simulink model "benchmark_model_2"  (R2021a)
settings: Solver=ode1  StartTime=0.0  StopTime=Tend  FixedStep=0.0001  MaxStep=0.1  MinStep=0.0001  AbsTol=0.01  EnableMultiTasking=on
values from neighbouring files (symbols this model uses):
  A1 = 0.00017774967488    [engine_data.mat]
  A2 = 740220.330082    [engine_data.mat]
  AL = [6 6.5 7 7.5 8 8.5 9 9.5 10 10.5 11 11.5 ... (33 elements, 33x1)]    [engine_data.mat]
  AM0 = 0.02884    [engine_data.mat]
  AREA = 0.00580880481649    [engine_data.mat]
  BORE = 0.086    [engine_data.mat]
  C_EGR = 1.5    [engine_data.mat]
  c_f = 800000    [engine_data.mat]
  c_T = 1    [engine_data.mat]
  CAIR = [0 0 0 0.21 0 0 0.79]    [engine_data.mat]
  cCO = 0    [engine_data.mat]
  cCO2 = 0    [engine_data.mat]
  cH2 = 0    [engine_data.mat]
  cH2O = 0    [engine_data.mat]
  cHC = 0    [engine_data.mat]
  cN2 = 0.79    [engine_data.mat]
  CO = [22.3416398376 20.8398063107 19.3759939408 17.9445472871 16.538827802 15.1528221174 13.7819470707 12.4234138404 11.076283262 9.74128071245 8.42044156849 7.11667724438 ... (33 elements, 33x1)]    [engine_data.mat]
  CO2 = [1.08016197936 1.63070203699 2.20578946805 2.80905596198 3.44329822989 4.11013545224 4.80975559522 5.54078746844 6.30033629562 7.08419123341 7.88717005398 8.70352822078 ... (33 elements, 33x1)]    [engine_data.mat]
  cO2 = 0.21    [engine_data.mat]
  DEN0 = 1.17881164668    [engine_data.mat]
  EGR_dia = 0.02    [engine_data.mat]
  EGR_sk = 0.125663706144    [engine_data.mat]
  EX_AREA = 0.00137444678595    [engine_data.mat]
  EX_M_AR = 0.0258532162804    [engine_data.mat]
  EXO = 40    [engine_data.mat]
  FD0 = 5    [engine_data.mat]
  FOM = [12 11.348 6.233 5 5.449 8.523 5]    [engine_data.mat]
  FR0 = 0    [engine_data.mat]
  FR_C1 = 305.731    [engine_data.mat]
  FR_C2 = 1.70183    [engine_data.mat]
  FR_C3 = 3188.7424    [engine_data.mat]
  FR_C4 = 0.000296028194151    [engine_data.mat]
  FR_C5 = 1.03    [engine_data.mat]
  H2 = [17.3855302766 15.0102176452 12.8820660449 10.9850020715 9.30240027035 7.81790027685 6.51548255669 5.37933989743 4.39378660966 3.5433012035 2.8127075229 2.1874445405 ... (33 elements, 33x1)]    [engine_data.mat]
  H2O = [3.81120036781 5.32559240945 6.64944794012 7.79700886885 8.78142378855 9.61507632366 10.310008356 10.8782622871 11.3320540899 11.6837509075 11.9456809954 12.1298414055 ... (33 elements, 33x1)]    [engine_data.mat]
  HC = [5481.3024964 4476.06435729 3754.34247414 3215.30411383 2799.83726136 2471.30975971 2205.97110777 1987.83348465 1805.78690133 1651.89669698 1520.35918152 1406.8402103 ... (33 elements, 33x1)]    [engine_data.mat]
  INC = 0    [engine_data.mat]
  INO = -40    [engine_data.mat]
  KET = 0.001    [engine_data.mat]
  Kex = 1.28224854645    [engine_data.mat]
  Kh = 0.00462    [engine_data.mat]
  MAS0 = 0.00471524658673    [engine_data.mat]
  MCh = 0.000588883862304    [engine_data.mat]
  MHC = 0.01383448    [engine_data.mat]
  MN2 = 0.028    [engine_data.mat]
  MO2 = 0.032    [engine_data.mat]
  MOLcylT = 0.00157069204711    [engine_data.mat]
  N2 = [54.5020363032 56.4529864816 58.2465252261 59.8999246568 61.4284172656 62.8453054261 64.1621746691 65.3891205654 66.5349581592 67.6074047194 68.6132342687 69.5584035698 ... (33 elements, 33x1)]    [engine_data.mat]
  O2 = [0.331300985803 0.293088680307 0.264743132617 0.242930742419 0.225648917415 0.211629427842 0.200034641439 0.190292592782 0.182002893523 0.174881554044 0.168729672297 0.163420998081 ... (33 elements, 33x1)]    [engine_data.mat]
  PR0 = 101324.72    [engine_data.mat]
  R150 = 157.079632679    [engine_data.mat]
  Rabs = 8.31441    [engine_data.mat]
  SPEC = [4 0.086 0.086 0.043 0.14665 14 1 0.1 0 0.5 0.005 0 ... (19 elements, 19x1)]    [engine_data.mat]
  TBORE = 0.055    [engine_data.mat]
  Tend = 120    [engine_data.mat]
  Th_HC = 0.1    [engine_data.mat]
  Th_knock = 0.401961937891    [engine_data.mat]
  THEX = [0 1 2 3 4 5 6 7 8 9 10 11 ... (721 elements, 1x721)]    [engine_data.mat]
  THIN = [0 1 2 3 4 5 6 7 8 9 10 11 ... (721 elements, 1x721)]    [engine_data.mat]
  TM0 = 298.15    [engine_data.mat]
  Tstart = 5    [engine_data.mat]
  TW0 = 353.15    [engine_data.mat]
  V_EX = 0.0001    [engine_data.mat]
  VAREX = [0 0 0 0 0 0 0 0 0 0 0 0 ... (721 elements, 1x721)]    [engine_data.mat]
  VARIN = [0 0 0 0 0 0 0 0 0 0 0 0 ... (721 elements, 1x721)]    [engine_data.mat]
  VH = 0.000499557214218    [engine_data.mat]
  VT = 3.84274780168e-05    [engine_data.mat]
  WOM = [0.01383448 0.04401 0.02801 0.032 0.002016 0.018016 0.028]    [engine_data.mat]
  y = 1.81    [engine_data.mat]
undefined symbols (not defined in the file or in its folder): DiscIntNeverNeededParam
libraries: pid_lib x3
(part 2 of 7)

== system benchmark_model_2/ENGINE/engine_s/cylinders/cyl3 ==
  In_state : Inport
  In_c : Inport  Port=2
  ex_state : Inport  Port=3
  ex_c : Inport  Port=4
  ECU_sa : Inport  Port=5
  ECU_fi : Inport  Port=6
  rps : Inport  Port=7
  st : Inport  Port=8
  EGR : Inport  Port=9
  in_vt : Inport  Port=10
  cyl : Subsystem
  ex_valve : Subsystem
  in_valve : Subsystem
  selectors : Subsystem
  af : Outport
  ex_fen : Outport  Port=2
  ex_fml : Outport  Port=3
  in_fen : Outport  Port=4
  in_fml : Outport  Port=5
  pc : Outport  Port=6
  QA : Outport  Port=7
  QR : Outport  Port=8
  KI : Outport  Port=9
  Knock : Outport  Port=10
  RHC : Outport  Port=11
  TR : Outport  Port=12
  sum_fc : Outport  Port=13
  fc : Outport  Port=14
  wires:
  rps/1 -> cyl/7(rps), selectors/7(rps)
  ECU_fi/1 -> selectors/6(ECU_fi)
  ECU_sa/1 -> selectors/5(ECU_sa)
  st/1 -> selectors/4(st)
  In_state/1 -> in_valve/5(u_st)
  ex_state/1 -> ex_valve/1(d_st)
  cyl/1(cyl_state) -> in_valve/2(d_st), ex_valve/4(u_st)
  cyl/2(cyl_c) -> ex_valve/5(u_c), in_valve/1(d_c)
  In_c/1 -> in_valve/6(u_c)
  selectors/1(ecu) -> ex_valve/3(ecu), in_valve/3(ecu), cyl/5(ecu)
  cyl/3(pc) -> pc/1
  ex_c/1 -> ex_valve/2(d_c)
  ex_valve/1(fen) -> cyl/1(ex_fen), ex_fen/1
  ex_valve/2(fml) -> cyl/2(ex_fml), ex_fml/1
  in_valve/1(fen) -> cyl/3(in_fen), in_fen/1
  in_valve/2(fml) -> cyl/4(in_fml), selectors/1(fml), in_fml/1
  cyl/4(af) -> af/1
  selectors/2(KL) -> cyl/6(KL)
  cyl/5(QA) -> QA/1
  cyl/6(QR) -> QR/1
  cyl/7(KI) -> KI/1
  in_valve/3(fms) -> selectors/2(fms)
  EGR/1 -> cyl/8(EGR)
  cyl/8(Knock) -> Knock/1
  cyl/9(R_HC) -> RHC/1
  in_vt/1 -> selectors/3(ECU_vt), in_valve/4(in_vt)
  cyl/10(TR) -> TR/1
  selectors/3(sum_fc) -> sum_fc/1
  selectors/4(fc) -> fc/1

== system benchmark_model_2/ENGINE/engine_s/cylinders/cyl4 ==
  In_state : Inport
  In_c : Inport  Port=2
  ex_state : Inport  Port=3
  ex_c : Inport  Port=4
  ECU_sa : Inport  Port=5
  ECU_fi : Inport  Port=6
  rps : Inport  Port=7
  st : Inport  Port=8
  EGR : Inport  Port=9
  in_vt : Inport  Port=10
  cyl : Subsystem
  ex_valve : Subsystem
  in_valve : Subsystem
  selectors : Subsystem
  af : Outport
  ex_fen : Outport  Port=2
  ex_fml : Outport  Port=3
  in_fen : Outport  Port=4
  in_fml : Outport  Port=5
  pc : Outport  Port=6
  QA : Outport  Port=7
  QR : Outport  Port=8
  KI : Outport  Port=9
  Knock : Outport  Port=10
  RHC : Outport  Port=11
  TR : Outport  Port=12
  sum_fc : Outport  Port=13
  fc : Outport  Port=14
  wires:
  selectors/3(sum_fc) -> sum_fc/1
  cyl/10(TR) -> TR/1
  in_vt/1 -> in_valve/4(in_vt), selectors/3(ECU_vt)
  cyl/9(R_HC) -> RHC/1
  cyl/8(Knock) -> Knock/1
  EGR/1 -> cyl/8(EGR)
  in_valve/3(fms) -> selectors/2(fms)
  cyl/7(KI) -> KI/1
  cyl/6(QR) -> QR/1
  cyl/5(QA) -> QA/1
  selectors/2(KL) -> cyl/6(KL)
  cyl/4(af) -> af/1
  in_valve/2(fml) -> in_fml/1, selectors/1(fml), cyl/4(in_fml)
  in_valve/1(fen) -> in_fen/1, cyl/3(in_fen)
  ex_valve/2(fml) -> ex_fml/1, cyl/2(ex_fml)
  ex_valve/1(fen) -> ex_fen/1, cyl/1(ex_fen)
  ex_c/1 -> ex_valve/2(d_c)
  cyl/3(pc) -> pc/1
  selectors/1(ecu) -> cyl/5(ecu), in_valve/3(ecu), ex_valve/3(ecu)
  In_c/1 -> in_valve/6(u_c)
  cyl/2(cyl_c) -> in_valve/1(d_c), ex_valve/5(u_c)
  cyl/1(cyl_state) -> ex_valve/4(u_st), in_valve/2(d_st)
  ex_state/1 -> ex_valve/1(d_st)
  In_state/1 -> in_valve/5(u_st)
  st/1 -> selectors/4(st)
  ECU_sa/1 -> selectors/5(ECU_sa)
  ECU_fi/1 -> selectors/6(ECU_fi)
  rps/1 -> selectors/7(rps), cyl/7(rps)
  selectors/4(fc) -> fc/1

== system benchmark_model_2/ENGINE/engine_s/ex_chamber/In_vol ==
  EGR_fen : Inport
  EGR_fml : Inport  Port=2
  out_fen : Inport  Port=3
  out_fml : Inport  Port=4
  in_fen : Inport  Port=5
  in_fml : Inport  Port=6
  Enrgy_Int : Subsystem
  Mol_Int : Subsystem
  cal_cyl_state : Subsystem
  V_temp : Outport  InitialOutput=0
  V_state : Outport  Port=2  InitialOutput=0
  V_c : Outport  Port=3  InitialOutput=0
  wires:
  cal_cyl_state/1(V_temp) -> Enrgy_Int/1(temp), V_temp/1
  out_fen/1 -> Enrgy_Int/3(Enrgy_out)
  in_fen/1 -> Enrgy_Int/2(Enrgy_In)
  out_fml/1 -> Mol_Int/2(nml_out)
  in_fml/1 -> Mol_Int/1(nml_In)
  Enrgy_Int/1(E) -> cal_cyl_state/1(E)
  Mol_Int/1(Nmol) -> cal_cyl_state/2(Nml)
  cal_cyl_state/2(V_st) -> V_state/1
  cal_cyl_state/3(V_c) -> V_c/1
  EGR_fen/1 -> Enrgy_Int/4(Enrgy_EGR)
  EGR_fml/1 -> Mol_Int/3(nml_EGR)

== system benchmark_model_2/ENGINE/engine_s/in_chamber/In_vol ==
  EGR_fen : Inport
  EGR_fml : Inport  Port=2
  out_fen : Inport  Port=3
  out_fml : Inport  Port=4
  in_fen : Inport  Port=5
  in_fml : Inport  Port=6
  Enrgy_Int : Subsystem
  Mol_Int : Subsystem
  cal_cyl_state : Subsystem
  C_signed_C : Outport  InitialOutput=0
  V_state : Outport  Port=2  InitialOutput=0
  V_c : Outport  Port=3  InitialOutput=0
  C_C : Outport  Port=4  InitialOutput=0
  wires:
  cal_cyl_state/2(V_c) -> V_c/1
  cal_cyl_state/1(V_st) -> V_state/1
  Mol_Int/1(Nmol) -> cal_cyl_state/2(Nml)
  Enrgy_Int/1(X_dens) -> cal_cyl_state/1(E)
  in_fml/1 -> Mol_Int/1(nml_In)
  out_fml/1 -> Mol_Int/2(nml_out)
  in_fen/1 -> Enrgy_Int/1(Enrgy_In)
  out_fen/1 -> Enrgy_Int/2(Enrgy_out)
  EGR_fen/1 -> Enrgy_Int/3(Enrgy_EGR)
  EGR_fml/1 -> Mol_Int/3(nml_EGR)
  Mol_Int/2(C_signed_C) -> C_signed_C/1
  Mol_Int/3(C_C) -> C_C/1

== system benchmark_model_2/ENGINE/engine_s/rpm_dynamics1/stroke ==
  CA : Inport
  Constant : Constant  Value=pi
  Mux : Mux
  Sum : Sum  Inputs=+-|  InputSameDT=on  SaturateOnIntegerOverflow=on  OutDataTypeStr=Inherit: Same as first input
  Sum1 : Sum  Inputs=+-|  InputSameDT=on  SaturateOnIntegerOverflow=on  OutDataTypeStr=Inherit: Same as first input
  Sum2 : Sum  Inputs=+-|  InputSameDT=on  SaturateOnIntegerOverflow=on  OutDataTypeStr=Inherit: Same as first input
  mod720(u,4*pi) : Subsystem
  mod720(u,4*pi)1 : Subsystem
  mod720(u,4*pi)2 : Subsystem
  mod720(u,4*pi)3 : Subsystem
  st(1-4) : Outport
  wires:
  CA/1 -> mod720(u,4*pi)/1(u), Sum/1
  mod720(u,4*pi)/1(y) -> Mux/1
  Mux/1 -> st(1-4)/1
  Sum2/1 -> mod720(u,4*pi)3/1(u)
  Constant/1 -> Sum1/2, Sum/2, Sum2/2
  Sum1/1 -> mod720(u,4*pi)2/1(u), Sum2/1
  Sum/1 -> mod720(u,4*pi)1/1(u), Sum1/1
  mod720(u,4*pi)1/1(y) -> Mux/3
  mod720(u,4*pi)2/1(y) -> Mux/4
  mod720(u,4*pi)3/1(y) -> Mux/2

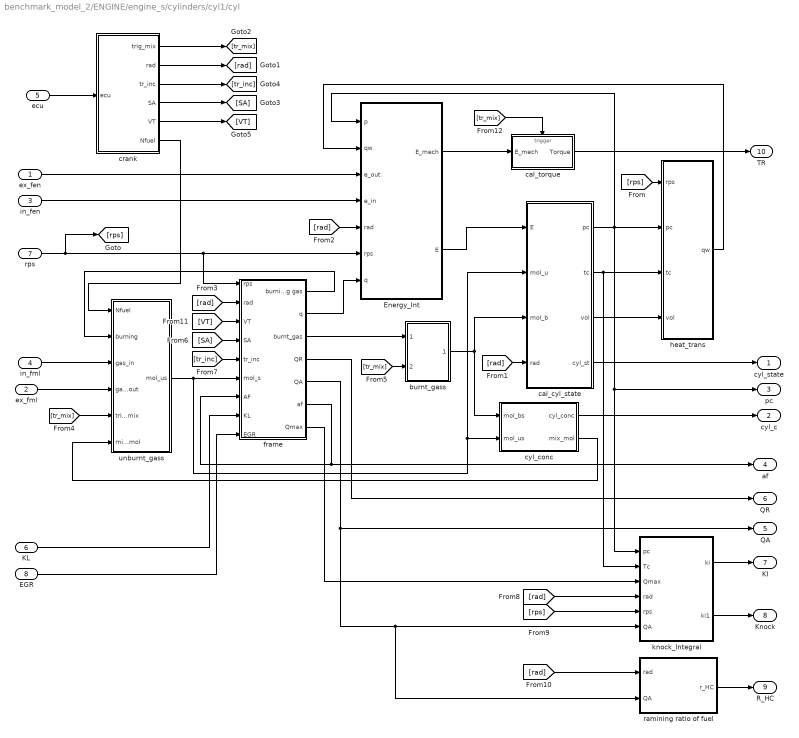
== system benchmark_model_2/ENGINE/engine_s/cylinders/cyl1/cyl ==
  ex_fen : Inport
  ex_fml : Inport  Port=2
  in_fen : Inport  Port=3
  in_fml : Inport  Port=4
  ecu : Inport  Port=5
  KL : Inport  Port=6
  rps : Inport  Port=7
  EGR : Inport  Port=8
  Energy_Int : Subsystem
  burnt_gass : Subsystem
  cal_cyl_state : Subsystem
  cal_torque : Subsystem
  crank : Subsystem
  cyl_conc : Subsystem
  frame : Subsystem
  heat_trans : Subsystem
  knock_Integral : Subsystem
  ramining ratio of fuel : Subsystem
  unburnt_gass : Subsystem
  cyl_state : Outport  InitialOutput=0
  cyl_c : Outport  Port=2  InitialOutput=0
  pc : Outport  Port=3  InitialOutput=0
  af : Outport  Port=4  InitialOutput=0
  QA : Outport  Port=5  InitialOutput=0
  QR : Outport  Port=6  InitialOutput=0
  KI : Outport  Port=7  InitialOutput=0
  Knock : Outport  Port=8  InitialOutput=0
  R_HC : Outport  Port=9  InitialOutput=0
  TR : Outport  Port=10  InitialOutput=0
  wires:
  heat_trans/1(qw) -> Energy_Int/2(qw)
  frame/2(q) -> Energy_Int/7(q)
  frame/3(burnt_gas) -> burnt_gass/1(gas_in)
  unburnt_gass/1(mol_us) -> cyl_conc/2(mol_us), cal_cyl_state/2(mol_u), frame/6(mol_s)
  rps/1 -> [rps], frame/1(rps), Energy_Int/6(rps)
  in_fml/1 -> unburnt_gass/3(gas_in)
  burnt_gass/1(mol_bs) -> cal_cyl_state/3(mol_b), cyl_conc/1(mol_bs)
  cyl_conc/1(cyl_conc) -> cyl_c/1
  [rps] -> heat_trans/1(rps)
  ecu/1 -> crank/1(ecu)
  [rad] -> Energy_Int/5(rad)
  [rad] -> frame/2(rad)
  ex_fen/1 -> Energy_Int/3(e_out)
  in_fen/1 -> Energy_Int/4(e_in)
  ex_fml/1 -> unburnt_gass/4(gas_out)
  frame/1(burning gas) -> unburnt_gass/2(burning)
  crank/1(trig_mix) -> [tr_mix]
  [tr_mix] -> unburnt_gass/5(trig_mix)
  [tr_mix] -> burnt_gass/2(tr_mix)
  crank/2(rad) -> [rad]
  frame/6(af) -> af/1, frame/7(AF)
  crank/6(Nfuel) -> unburnt_gass/1(Nfuel)
  [tr_inc] -> frame/5(tr_inc)
  cyl_conc/2(mix_mol) -> unburnt_gass/6(mix_mol)
  crank/3(tr_inc) -> [tr_inc]
  cal_cyl_state/1(pc) -> heat_trans/2(pc), Energy_Int/1(p), pc/1, knock_Integral/1(pc)
  [rad] -> cal_cyl_state/4(rad)
  cal_cyl_state/4(cyl_st) -> cyl_state/1
  cal_cyl_state/3(vol) -> heat_trans/4(vol)
  cal_cyl_state/2(tc) -> knock_Integral/2(Tc), heat_trans/3(tc)
  Energy_Int/2(E) -> cal_cyl_state/1(E)
  crank/4(SA) -> [SA]
  [SA] -> frame/4(SA)
  KL/1 -> frame/8(KL)
  frame/4(QR) -> QR/1
  knock_Integral/1(ki) -> KI/1
  EGR/1 -> frame/9(EGR)
  [rad] -> knock_Integral/4(rad)
  frame/5(QA) -> QA/1, ramining ratio of fuel/2(QA), knock_Integral/6(QA)
  [rps] -> knock_Integral/5(rps)
  knock_Integral/2(ki1) -> Knock/1
  [rad] -> ramining ratio of fuel/1(rad)
  ramining ratio of fuel/1(r_HC) -> R_HC/1
  frame/7(Qmax) -> knock_Integral/3(Qmax)
  [VT] -> frame/3(VT)
  crank/5(VT) -> [VT]
  Energy_Int/1(E_mech) -> cal_torque/1(E_mech)
  cal_torque/1(Torque) -> TR/1
  [tr_mix] -> cal_torque/Trigger

== system benchmark_model_2/ENGINE/engine_s/cylinders/cyl1/ex_valve ==
  d_st : Inport
  d_c : Inport  Port=2
  ecu : Inport  Port=3
  u_st : Inport  Port=4  PortDimensions=4
  u_c : Inport  Port=5
  Constant : Constant  Value=WOM
  Constant1 : Constant  Value=4*pi
  Gain : Gain  Gain=180/pi
  Lookup Table1 : Lookup  InputValues=THEX  Table=VAREX
  Math Function : Math  Operator=mod  SignedPower=on  SaturateOnIntegerOverflow=on
  Selector : Selector  InputPortWidth=6  IndexOptions=Index vector (dialog)  Indices=1  OutputSizes=[(-2)]
  cal_flow : MATLAB Function  TreatAsAtomicUnit=on
  fen : Outport  PortDimensions=1
  fml : Outport  Port=2  PortDimensions=7
  wires:
  ecu/1 -> Selector/1
  cal_flow/1(fen) -> fen/1
  Lookup Table1/1 -> cal_flow/1(area)
  u_st/1 -> cal_flow/2(inlet)
  u_c/1 -> cal_flow/3(c_in)
  d_st/1 -> cal_flow/4(outlet)
  d_c/1 -> cal_flow/5(c_out)
  cal_flow/2(fml) -> fml/1
  Constant/1 -> cal_flow/6(WOM)
  Gain/1 -> Lookup Table1/1
  Math Function/1 -> Gain/1
  Selector/1 -> Math Function/1
  Constant1/1 -> Math Function/2

== system benchmark_model_2/ENGINE/engine_s/cylinders/cyl1/in_valve ==
  d_c : Inport
  d_st : Inport  Port=2
  ecu : Inport  Port=3
  in_vt : Inport  Port=4
  u_st : Inport  Port=5
  u_c : Inport  Port=6
  Add : Sum  Inputs=-+
  Constant : Constant  Value=WOM
  Gain : Gain  Gain=180/pi
  Lookup Table : Lookup  InputValues=THIN  Table=VARIN
  Selector1 : Selector  InputPortWidth=6  IndexOptions=Index vector (dialog)  Indices=1  OutputSizes=[(-2)]
  cal_flow : MATLAB Function  TreatAsAtomicUnit=on
  fen : Outport  PortDimensions=1
  fml : Outport  Port=2  PortDimensions=7
  fms : Outport  Port=3  PortDimensions=1
  wires:
  Gain/1 -> Lookup Table/1
  ecu/1 -> Selector1/1
  u_st/1 -> cal_flow/2(inlet)
  Lookup Table/1 -> cal_flow/1(area)
  d_st/1 -> cal_flow/4(outlet)
  cal_flow/1(fen) -> fen/1
  u_c/1 -> cal_flow/3(c_in)
  d_c/1 -> cal_flow/5(c_out)
  cal_flow/2(fml) -> fml/1
  cal_flow/3(fms) -> fms/1
  Constant/1 -> cal_flow/6(WOM)
  in_vt/1 -> Add/1
  Selector1/1 -> Add/2
  Add/1 -> Gain/1

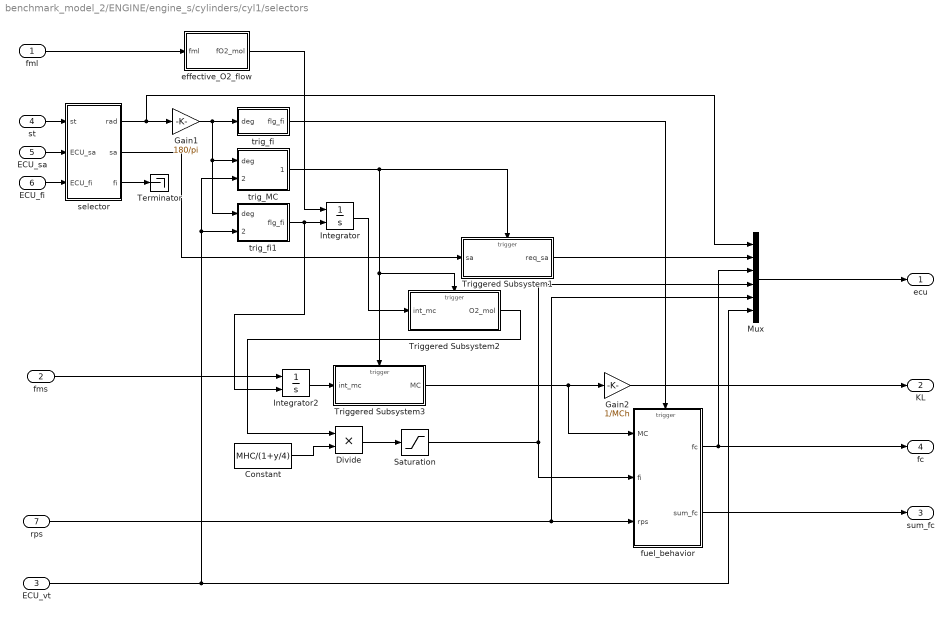
== system benchmark_model_2/ENGINE/engine_s/cylinders/cyl1/selectors ==
  fml : Inport
  fms : Inport  Port=2
  ECU_vt : Inport  Port=3
  st : Inport  Port=4
  ECU_sa : Inport  Port=5
  ECU_fi : Inport  Port=6
  rps : Inport  Port=7
  Constant : Constant  Value=MHC/(1+y/4)
  Divide : Product
  Gain1 : Gain  Gain=180/pi
  Gain2 : Gain  Gain=1/MCh
  Integrator : Integrator  ExternalReset=rising
  Integrator2 : Integrator  ExternalReset=rising
  Mux : Mux  Inputs=6
  Saturation : Saturate  UpperLimit=inf  LowerLimit=0
  Terminator : Terminator
  Triggered Subsystem1 : Subsystem  TreatAsAtomicUnit=on
  Triggered Subsystem2 : Subsystem  TreatAsAtomicUnit=on
  Triggered Subsystem3 : Subsystem  TreatAsAtomicUnit=on
  effective_O2_flow : Subsystem
  fuel_behavior : Subsystem  TreatAsAtomicUnit=on
  selector : Subsystem
  trig_MC : Subsystem
  trig_fi : Subsystem
  trig_fi1 : Subsystem
  ecu : Outport
  KL : Outport  Port=2
  sum_fc : Outport  Port=3
  fc : Outport  Port=4
  wires:
  Triggered Subsystem2/1(O2_mol) -> Divide/1
  Gain1/1 -> trig_fi/1(deg), trig_fi1/1(deg), trig_MC/1(deg)
  ECU_fi/1 -> selector/3(ECU_fi)
  ECU_sa/1 -> selector/2(ECU_sa)
  st/1 -> selector/1(st)
  trig_MC/1(flg_inc) -> Triggered Subsystem3/Trigger, Triggered Subsystem2/Trigger, Triggered Subsystem1/Trigger
  rps/1 -> Mux/5, fuel_behavior/3(rps)
  selector/1(rad) -> Gain1/1, Mux/1
  Mux/1 -> ecu/1
  trig_fi/1(flg_fi) -> fuel_behavior/Trigger
  selector/2(sa) -> Triggered Subsystem1/1(sa)
  Triggered Subsystem1/1(req_sa) -> Mux/2
  trig_fi1/1(flg_fi) -> Integrator/2, Integrator2/2
  Integrator/1 -> Triggered Subsystem2/1(int_mc)
  fuel_behavior/1(fc) -> fc/1, Mux/3
  selector/3(fi) -> Terminator/1
  Gain2/1 -> KL/1
  Divide/1 -> Saturation/1
  fml/1 -> effective_O2_flow/1(fml)
  effective_O2_flow/1(fO2_mol) -> Integrator/1
  Constant/1 -> Divide/2
  Saturation/1 -> fuel_behavior/2(fi), Mux/4
  Integrator2/1 -> Triggered Subsystem3/1(int_mc)
  Triggered Subsystem3/1(MC) -> Gain2/1, fuel_behavior/1(MC)
  fms/1 -> Integrator2/1
  ECU_vt/1 -> trig_MC/2(ECU_vvt), trig_fi1/2(ECU_vvt), Mux/6
  fuel_behavior/2(sum_fc) -> sum_fc/1

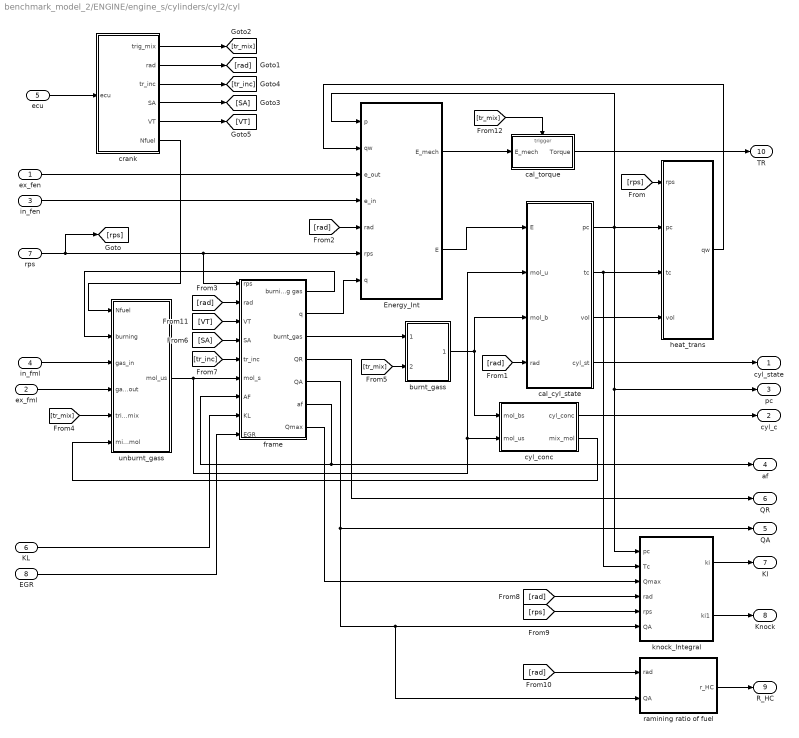
== system benchmark_model_2/ENGINE/engine_s/cylinders/cyl2/cyl ==
  ex_fen : Inport
  ex_fml : Inport  Port=2
  in_fen : Inport  Port=3
  in_fml : Inport  Port=4
  ecu : Inport  Port=5
  KL : Inport  Port=6
  rps : Inport  Port=7
  EGR : Inport  Port=8
  Energy_Int : Subsystem
  burnt_gass : Subsystem
  cal_cyl_state : Subsystem
  cal_torque : Subsystem
  crank : Subsystem
  cyl_conc : Subsystem
  frame : Subsystem
  heat_trans : Subsystem
  knock_Integral : Subsystem
  ramining ratio of fuel : Subsystem
  unburnt_gass : Subsystem
  cyl_state : Outport  InitialOutput=0
  cyl_c : Outport  Port=2  InitialOutput=0
  pc : Outport  Port=3  InitialOutput=0
  af : Outport  Port=4  InitialOutput=0
  QA : Outport  Port=5  InitialOutput=0
  QR : Outport  Port=6  InitialOutput=0
  KI : Outport  Port=7  InitialOutput=0
  Knock : Outport  Port=8  InitialOutput=0
  R_HC : Outport  Port=9  InitialOutput=0
  TR : Outport  Port=10  InitialOutput=0
  wires:
  [tr_mix] -> cal_torque/Trigger
  cal_torque/1(Torque) -> TR/1
  Energy_Int/1(E_mech) -> cal_torque/1(E_mech)
  crank/5(VT) -> [VT]
  [VT] -> frame/3(VT)
  frame/7(Qmax) -> knock_Integral/3(Qmax)
  ramining ratio of fuel/1(r_HC) -> R_HC/1
  [rad] -> ramining ratio of fuel/1(rad)
  knock_Integral/2(ki1) -> Knock/1
  [rps] -> knock_Integral/5(rps)
  frame/5(QA) -> knock_Integral/6(QA), ramining ratio of fuel/2(QA), QA/1
  [rad] -> knock_Integral/4(rad)
  EGR/1 -> frame/9(EGR)
  knock_Integral/1(ki) -> KI/1
  frame/4(QR) -> QR/1
  KL/1 -> frame/8(KL)
  [SA] -> frame/4(SA)
  crank/4(SA) -> [SA]
  Energy_Int/2(E) -> cal_cyl_state/1(E)
  cal_cyl_state/2(tc) -> heat_trans/3(tc), knock_Integral/2(Tc)
  cal_cyl_state/3(vol) -> heat_trans/4(vol)
  cal_cyl_state/4(cyl_st) -> cyl_state/1
  [rad] -> cal_cyl_state/4(rad)
  cal_cyl_state/1(pc) -> knock_Integral/1(pc), pc/1, Energy_Int/1(p), heat_trans/2(pc)
  crank/3(tr_inc) -> [tr_inc]
  cyl_conc/2(mix_mol) -> unburnt_gass/6(mix_mol)
  [tr_inc] -> frame/5(tr_inc)
  crank/6(Nfuel) -> unburnt_gass/1(Nfuel)
  frame/6(af) -> frame/7(AF), af/1
  crank/2(rad) -> [rad]
  [tr_mix] -> burnt_gass/2(tr_mix)
  [tr_mix] -> unburnt_gass/5(trig_mix)
  crank/1(trig_mix) -> [tr_mix]
  frame/1(burning gas) -> unburnt_gass/2(burning)
  ex_fml/1 -> unburnt_gass/4(gas_out)
  in_fen/1 -> Energy_Int/4(e_in)
  ex_fen/1 -> Energy_Int/3(e_out)
  [rad] -> frame/2(rad)
  [rad] -> Energy_Int/5(rad)
  ecu/1 -> crank/1(ecu)
  [rps] -> heat_trans/1(rps)
  cyl_conc/1(cyl_conc) -> cyl_c/1
  burnt_gass/1(mol_bs) -> cyl_conc/1(mol_bs), cal_cyl_state/3(mol_b)
  in_fml/1 -> unburnt_gass/3(gas_in)
  rps/1 -> Energy_Int/6(rps), frame/1(rps), [rps]
  unburnt_gass/1(mol_us) -> frame/6(mol_s), cal_cyl_state/2(mol_u), cyl_conc/2(mol_us)
  frame/3(burnt_gas) -> burnt_gass/1(gas_in)
  frame/2(q) -> Energy_Int/7(q)
  heat_trans/1(qw) -> Energy_Int/2(qw)

== system benchmark_model_2/ENGINE/engine_s/cylinders/cyl2/ex_valve ==
  d_st : Inport
  d_c : Inport  Port=2
  ecu : Inport  Port=3
  u_st : Inport  Port=4  PortDimensions=4
  u_c : Inport  Port=5
  Constant : Constant  Value=WOM
  Constant1 : Constant  Value=4*pi
  Gain : Gain  Gain=180/pi
  Lookup Table1 : Lookup  InputValues=THEX  Table=VAREX
  Math Function : Math  Operator=mod  SignedPower=on  SaturateOnIntegerOverflow=on
  Selector : Selector  InputPortWidth=6  IndexOptions=Index vector (dialog)  Indices=1  OutputSizes=[(-2)]
  cal_flow : MATLAB Function  TreatAsAtomicUnit=on
  fen : Outport  PortDimensions=1
  fml : Outport  Port=2  PortDimensions=7
  wires:
  Constant1/1 -> Math Function/2
  Selector/1 -> Math Function/1
  Math Function/1 -> Gain/1
  Gain/1 -> Lookup Table1/1
  Constant/1 -> cal_flow/6(WOM)
  cal_flow/2(fml) -> fml/1
  d_c/1 -> cal_flow/5(c_out)
  d_st/1 -> cal_flow/4(outlet)
  u_c/1 -> cal_flow/3(c_in)
  u_st/1 -> cal_flow/2(inlet)
  Lookup Table1/1 -> cal_flow/1(area)
  cal_flow/1(fen) -> fen/1
  ecu/1 -> Selector/1

== system benchmark_model_2/ENGINE/engine_s/cylinders/cyl2/in_valve ==
  d_c : Inport
  d_st : Inport  Port=2
  ecu : Inport  Port=3
  in_vt : Inport  Port=4
  u_st : Inport  Port=5
  u_c : Inport  Port=6
  Add : Sum  Inputs=-+
  Constant : Constant  Value=WOM
  Gain : Gain  Gain=180/pi
  Lookup Table : Lookup  InputValues=THIN  Table=VARIN
  Selector1 : Selector  InputPortWidth=6  IndexOptions=Index vector (dialog)  Indices=1  OutputSizes=[(-2)]
  cal_flow : MATLAB Function  TreatAsAtomicUnit=on
  fen : Outport  PortDimensions=1
  fml : Outport  Port=2  PortDimensions=7
  fms : Outport  Port=3  PortDimensions=1
  wires:
  Add/1 -> Gain/1
  Selector1/1 -> Add/2
  in_vt/1 -> Add/1
  Constant/1 -> cal_flow/6(WOM)
  cal_flow/3(fms) -> fms/1
  cal_flow/2(fml) -> fml/1
  d_c/1 -> cal_flow/5(c_out)
  u_c/1 -> cal_flow/3(c_in)
  cal_flow/1(fen) -> fen/1
  d_st/1 -> cal_flow/4(outlet)
  Lookup Table/1 -> cal_flow/1(area)
  u_st/1 -> cal_flow/2(inlet)
  ecu/1 -> Selector1/1
  Gain/1 -> Lookup Table/1

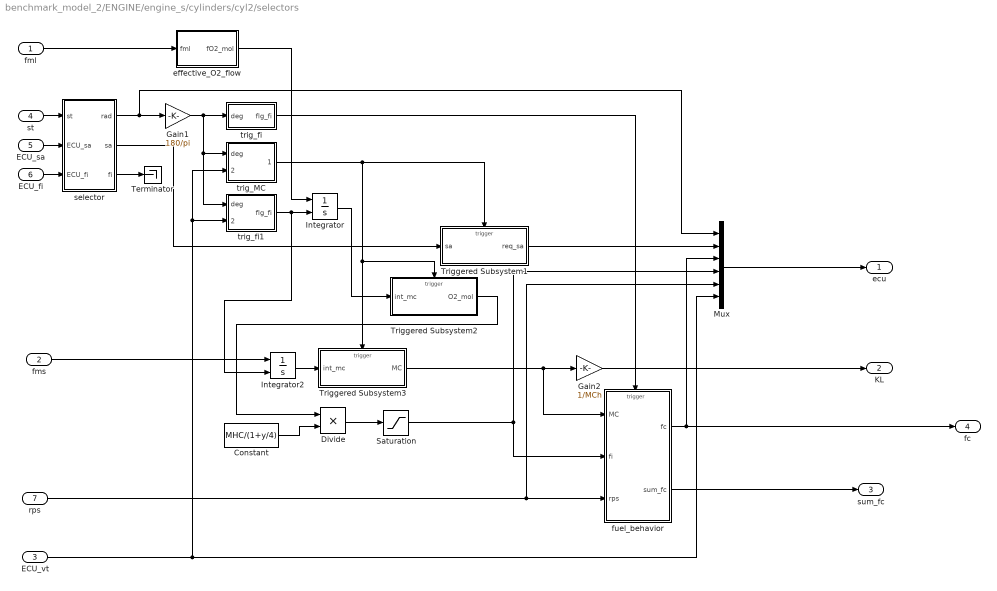
== system benchmark_model_2/ENGINE/engine_s/cylinders/cyl2/selectors ==
  fml : Inport
  fms : Inport  Port=2
  ECU_vt : Inport  Port=3
  st : Inport  Port=4
  ECU_sa : Inport  Port=5
  ECU_fi : Inport  Port=6
  rps : Inport  Port=7
  Constant : Constant  Value=MHC/(1+y/4)
  Divide : Product
  Gain1 : Gain  Gain=180/pi
  Gain2 : Gain  Gain=1/MCh
  Integrator : Integrator  ExternalReset=rising
  Integrator2 : Integrator  ExternalReset=rising
  Mux : Mux  Inputs=6
  Saturation : Saturate  UpperLimit=inf  LowerLimit=0
  Terminator : Terminator
  Triggered Subsystem1 : Subsystem  TreatAsAtomicUnit=on
  Triggered Subsystem2 : Subsystem  TreatAsAtomicUnit=on
  Triggered Subsystem3 : Subsystem  TreatAsAtomicUnit=on
  effective_O2_flow : Subsystem
  fuel_behavior : Subsystem  TreatAsAtomicUnit=on
  selector : Subsystem
  trig_MC : Subsystem
  trig_fi : Subsystem
  trig_fi1 : Subsystem
  ecu : Outport
  KL : Outport  Port=2
  sum_fc : Outport  Port=3
  fc : Outport  Port=4
  wires:
  fuel_behavior/2(sum_fc) -> sum_fc/1
  ECU_vt/1 -> Mux/6, trig_fi1/2(ECU_vvt), trig_MC/2(ECU_vvt)
  fms/1 -> Integrator2/1
  Triggered Subsystem3/1(MC) -> fuel_behavior/1(MC), Gain2/1
  Integrator2/1 -> Triggered Subsystem3/1(int_mc)
  Saturation/1 -> Mux/4, fuel_behavior/2(fi)
  Constant/1 -> Divide/2
  effective_O2_flow/1(fO2_mol) -> Integrator/1
  fml/1 -> effective_O2_flow/1(fml)
  Divide/1 -> Saturation/1
  Gain2/1 -> KL/1
  selector/3(fi) -> Terminator/1
  Integrator/1 -> Triggered Subsystem2/1(int_mc)
  trig_fi1/1(flg_fi) -> Integrator2/2, Integrator/2
  Triggered Subsystem1/1(req_sa) -> Mux/2
  selector/2(sa) -> Triggered Subsystem1/1(sa)
  trig_fi/1(flg_fi) -> fuel_behavior/Trigger
  Mux/1 -> ecu/1
  selector/1(rad) -> Mux/1, Gain1/1
  rps/1 -> fuel_behavior/3(rps), Mux/5
  trig_MC/1(flg_inc) -> Triggered Subsystem1/Trigger, Triggered Subsystem2/Trigger, Triggered Subsystem3/Trigger
  st/1 -> selector/1(st)
  ECU_sa/1 -> selector/2(ECU_sa)
  ECU_fi/1 -> selector/3(ECU_fi)
  Gain1/1 -> trig_MC/1(deg), trig_fi1/1(deg), trig_fi/1(deg)
  Triggered Subsystem2/1(O2_mol) -> Divide/1
  fuel_behavior/1(fc) -> fc/1, Mux/3

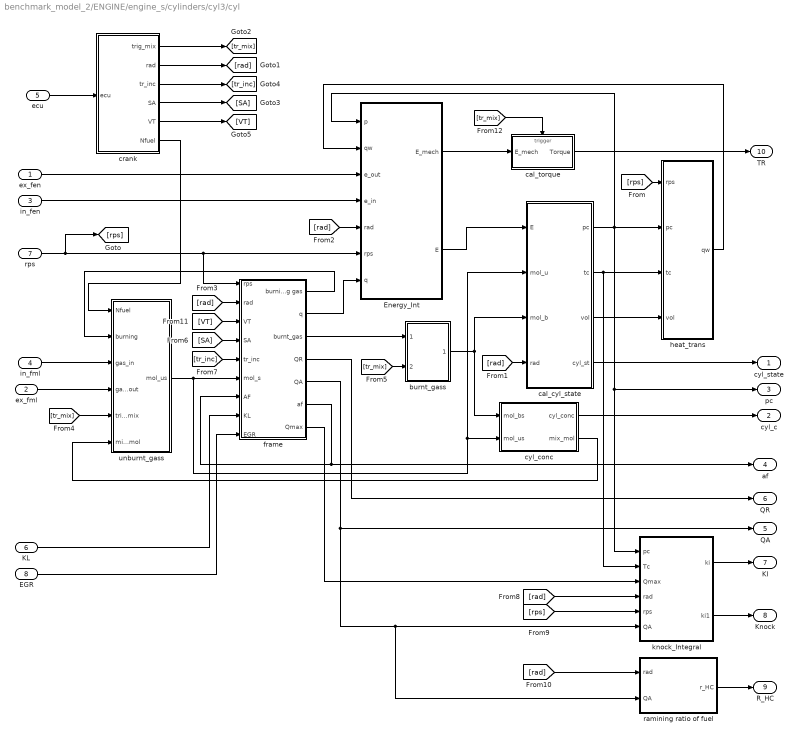
== system benchmark_model_2/ENGINE/engine_s/cylinders/cyl3/cyl ==
  ex_fen : Inport
  ex_fml : Inport  Port=2
  in_fen : Inport  Port=3
  in_fml : Inport  Port=4
  ecu : Inport  Port=5
  KL : Inport  Port=6
  rps : Inport  Port=7
  EGR : Inport  Port=8
  Energy_Int : Subsystem
  burnt_gass : Subsystem
  cal_cyl_state : Subsystem
  cal_torque : Subsystem
  crank : Subsystem
  cyl_conc : Subsystem
  frame : Subsystem
  heat_trans : Subsystem
  knock_Integral : Subsystem
  ramining ratio of fuel : Subsystem
  unburnt_gass : Subsystem
  cyl_state : Outport  InitialOutput=0
  cyl_c : Outport  Port=2  InitialOutput=0
  pc : Outport  Port=3  InitialOutput=0
  af : Outport  Port=4  InitialOutput=0
  QA : Outport  Port=5  InitialOutput=0
  QR : Outport  Port=6  InitialOutput=0
  KI : Outport  Port=7  InitialOutput=0
  Knock : Outport  Port=8  InitialOutput=0
  R_HC : Outport  Port=9  InitialOutput=0
  TR : Outport  Port=10  InitialOutput=0
  wires:
  heat_trans/1(qw) -> Energy_Int/2(qw)
  frame/2(q) -> Energy_Int/7(q)
  frame/3(burnt_gas) -> burnt_gass/1(gas_in)
  unburnt_gass/1(mol_us) -> cyl_conc/2(mol_us), cal_cyl_state/2(mol_u), frame/6(mol_s)
  rps/1 -> [rps], frame/1(rps), Energy_Int/6(rps)
  in_fml/1 -> unburnt_gass/3(gas_in)
  burnt_gass/1(mol_bs) -> cal_cyl_state/3(mol_b), cyl_conc/1(mol_bs)
  cyl_conc/1(cyl_conc) -> cyl_c/1
  [rps] -> heat_trans/1(rps)
  ecu/1 -> crank/1(ecu)
  [rad] -> Energy_Int/5(rad)
  [rad] -> frame/2(rad)
  ex_fen/1 -> Energy_Int/3(e_out)
  in_fen/1 -> Energy_Int/4(e_in)
  ex_fml/1 -> unburnt_gass/4(gas_out)
  frame/1(burning gas) -> unburnt_gass/2(burning)
  crank/1(trig_mix) -> [tr_mix]
  [tr_mix] -> unburnt_gass/5(trig_mix)
  [tr_mix] -> burnt_gass/2(tr_mix)
  crank/2(rad) -> [rad]
  frame/6(af) -> af/1, frame/7(AF)
  crank/6(Nfuel) -> unburnt_gass/1(Nfuel)
  [tr_inc] -> frame/5(tr_inc)
  cyl_conc/2(mix_mol) -> unburnt_gass/6(mix_mol)
  crank/3(tr_inc) -> [tr_inc]
  cal_cyl_state/1(pc) -> heat_trans/2(pc), Energy_Int/1(p), pc/1, knock_Integral/1(pc)
  [rad] -> cal_cyl_state/4(rad)
  cal_cyl_state/4(cyl_st) -> cyl_state/1
  cal_cyl_state/3(vol) -> heat_trans/4(vol)
  cal_cyl_state/2(tc) -> knock_Integral/2(Tc), heat_trans/3(tc)
  Energy_Int/2(E) -> cal_cyl_state/1(E)
  crank/4(SA) -> [SA]
  [SA] -> frame/4(SA)
  KL/1 -> frame/8(KL)
  frame/4(QR) -> QR/1
  knock_Integral/1(ki) -> KI/1
  EGR/1 -> frame/9(EGR)
  [rad] -> knock_Integral/4(rad)
  frame/5(QA) -> QA/1, ramining ratio of fuel/2(QA), knock_Integral/6(QA)
  [rps] -> knock_Integral/5(rps)
  knock_Integral/2(ki1) -> Knock/1
  [rad] -> ramining ratio of fuel/1(rad)
  ramining ratio of fuel/1(r_HC) -> R_HC/1
  frame/7(Qmax) -> knock_Integral/3(Qmax)
  [VT] -> frame/3(VT)
  crank/5(VT) -> [VT]
  Energy_Int/1(E_mech) -> cal_torque/1(E_mech)
  cal_torque/1(Torque) -> TR/1
  [tr_mix] -> cal_torque/Trigger

== system benchmark_model_2/ENGINE/engine_s/cylinders/cyl3/ex_valve ==
  d_st : Inport
  d_c : Inport  Port=2
  ecu : Inport  Port=3
  u_st : Inport  Port=4  PortDimensions=4
  u_c : Inport  Port=5
  Constant : Constant  Value=WOM
  Constant1 : Constant  Value=4*pi
  Gain : Gain  Gain=180/pi
  Lookup Table1 : Lookup  InputValues=THEX  Table=VAREX
  Math Function : Math  Operator=mod  SignedPower=on  SaturateOnIntegerOverflow=on
  Selector : Selector  InputPortWidth=6  IndexOptions=Index vector (dialog)  Indices=1  OutputSizes=[(-2)]
  cal_flow : MATLAB Function  TreatAsAtomicUnit=on
  fen : Outport  PortDimensions=1
  fml : Outport  Port=2  PortDimensions=7
  wires:
  ecu/1 -> Selector/1
  cal_flow/1(fen) -> fen/1
  Lookup Table1/1 -> cal_flow/1(area)
  u_st/1 -> cal_flow/2(inlet)
  u_c/1 -> cal_flow/3(c_in)
  d_st/1 -> cal_flow/4(outlet)
  d_c/1 -> cal_flow/5(c_out)
  cal_flow/2(fml) -> fml/1
  Constant/1 -> cal_flow/6(WOM)
  Gain/1 -> Lookup Table1/1
  Math Function/1 -> Gain/1
  Selector/1 -> Math Function/1
  Constant1/1 -> Math Function/2

== system benchmark_model_2/ENGINE/engine_s/cylinders/cyl3/in_valve ==
  d_c : Inport
  d_st : Inport  Port=2
  ecu : Inport  Port=3
  in_vt : Inport  Port=4
  u_st : Inport  Port=5
  u_c : Inport  Port=6
  Add : Sum  Inputs=-+
  Constant : Constant  Value=WOM
  Gain : Gain  Gain=180/pi
  Lookup Table : Lookup  InputValues=THIN  Table=VARIN
  Selector1 : Selector  InputPortWidth=6  IndexOptions=Index vector (dialog)  Indices=1  OutputSizes=[(-2)]
  cal_flow : MATLAB Function  TreatAsAtomicUnit=on
  fen : Outport  PortDimensions=1
  fml : Outport  Port=2  PortDimensions=7
  fms : Outport  Port=3  PortDimensions=1
  wires:
  Gain/1 -> Lookup Table/1
  ecu/1 -> Selector1/1
  u_st/1 -> cal_flow/2(inlet)
  Lookup Table/1 -> cal_flow/1(area)
  d_st/1 -> cal_flow/4(outlet)
  cal_flow/1(fen) -> fen/1
  u_c/1 -> cal_flow/3(c_in)
  d_c/1 -> cal_flow/5(c_out)
  cal_flow/2(fml) -> fml/1
  cal_flow/3(fms) -> fms/1
  Constant/1 -> cal_flow/6(WOM)
  in_vt/1 -> Add/1
  Selector1/1 -> Add/2
  Add/1 -> Gain/1

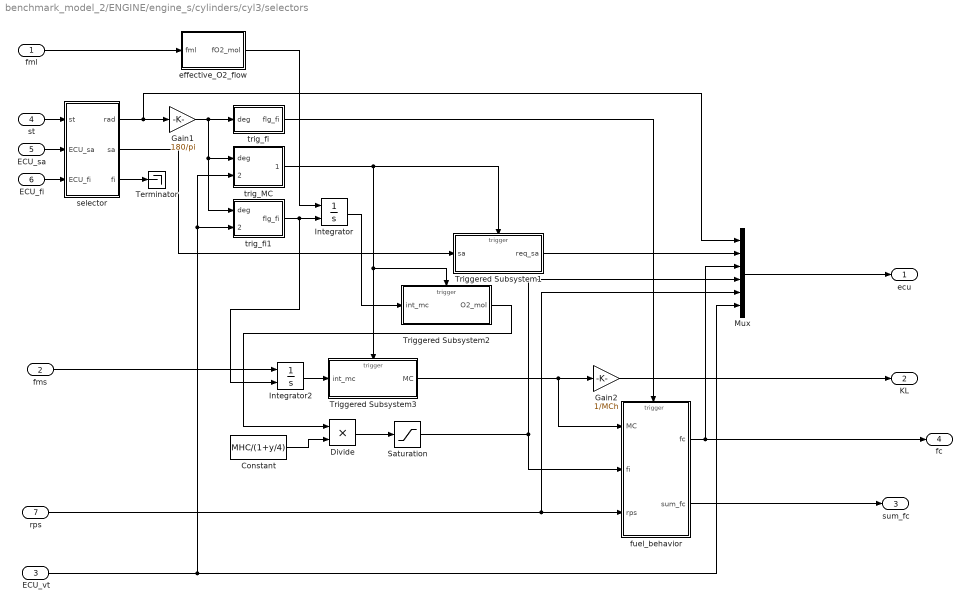
== system benchmark_model_2/ENGINE/engine_s/cylinders/cyl3/selectors ==
  fml : Inport
  fms : Inport  Port=2
  ECU_vt : Inport  Port=3
  st : Inport  Port=4
  ECU_sa : Inport  Port=5
  ECU_fi : Inport  Port=6
  rps : Inport  Port=7
  Constant : Constant  Value=MHC/(1+y/4)
  Divide : Product
  Gain1 : Gain  Gain=180/pi
  Gain2 : Gain  Gain=1/MCh
  Integrator : Integrator  ExternalReset=rising
  Integrator2 : Integrator  ExternalReset=rising
  Mux : Mux  Inputs=6
  Saturation : Saturate  UpperLimit=inf  LowerLimit=0
  Terminator : Terminator
  Triggered Subsystem1 : Subsystem  TreatAsAtomicUnit=on
  Triggered Subsystem2 : Subsystem  TreatAsAtomicUnit=on
  Triggered Subsystem3 : Subsystem  TreatAsAtomicUnit=on
  effective_O2_flow : Subsystem
  fuel_behavior : Subsystem  TreatAsAtomicUnit=on
  selector : Subsystem
  trig_MC : Subsystem
  trig_fi : Subsystem
  trig_fi1 : Subsystem
  ecu : Outport
  KL : Outport  Port=2
  sum_fc : Outport  Port=3
  fc : Outport  Port=4
  wires:
  Triggered Subsystem2/1(O2_mol) -> Divide/1
  Gain1/1 -> trig_fi/1(deg), trig_fi1/1(deg), trig_MC/1(deg)
  ECU_fi/1 -> selector/3(ECU_fi)
  ECU_sa/1 -> selector/2(ECU_sa)
  st/1 -> selector/1(st)
  trig_MC/1(flg_inc) -> Triggered Subsystem3/Trigger, Triggered Subsystem2/Trigger, Triggered Subsystem1/Trigger
  rps/1 -> Mux/5, fuel_behavior/3(rps)
  selector/1(rad) -> Gain1/1, Mux/1
  Mux/1 -> ecu/1
  trig_fi/1(flg_fi) -> fuel_behavior/Trigger
  selector/2(sa) -> Triggered Subsystem1/1(sa)
  Triggered Subsystem1/1(req_sa) -> Mux/2
  trig_fi1/1(flg_fi) -> Integrator/2, Integrator2/2
  Integrator/1 -> Triggered Subsystem2/1(int_mc)
  selector/3(fi) -> Terminator/1
  Gain2/1 -> KL/1
  Divide/1 -> Saturation/1
  fml/1 -> effective_O2_flow/1(fml)
  effective_O2_flow/1(fO2_mol) -> Integrator/1
  Constant/1 -> Divide/2
  Saturation/1 -> fuel_behavior/2(fi), Mux/4
  Integrator2/1 -> Triggered Subsystem3/1(int_mc)
  Triggered Subsystem3/1(MC) -> Gain2/1, fuel_behavior/1(MC)
  fms/1 -> Integrator2/1
  ECU_vt/1 -> trig_MC/2(ECU_vvt), trig_fi1/2(ECU_vvt), Mux/6
  fuel_behavior/2(sum_fc) -> sum_fc/1
  fuel_behavior/1(fc) -> fc/1, Mux/3

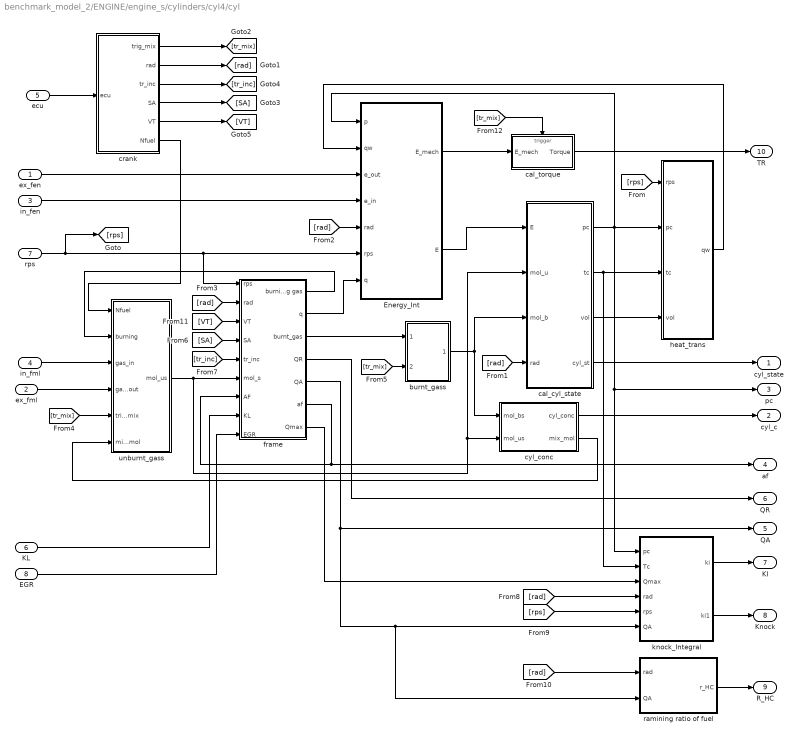
== system benchmark_model_2/ENGINE/engine_s/cylinders/cyl4/cyl ==
  ex_fen : Inport
  ex_fml : Inport  Port=2
  in_fen : Inport  Port=3
  in_fml : Inport  Port=4
  ecu : Inport  Port=5
  KL : Inport  Port=6
  rps : Inport  Port=7
  EGR : Inport  Port=8
  Energy_Int : Subsystem
  burnt_gass : Subsystem
  cal_cyl_state : Subsystem
  cal_torque : Subsystem
  crank : Subsystem
  cyl_conc : Subsystem
  frame : Subsystem
  heat_trans : Subsystem
  knock_Integral : Subsystem
  ramining ratio of fuel : Subsystem
  unburnt_gass : Subsystem
  cyl_state : Outport  InitialOutput=0
  cyl_c : Outport  Port=2  InitialOutput=0
  pc : Outport  Port=3  InitialOutput=0
  af : Outport  Port=4  InitialOutput=0
  QA : Outport  Port=5  InitialOutput=0
  QR : Outport  Port=6  InitialOutput=0
  KI : Outport  Port=7  InitialOutput=0
  Knock : Outport  Port=8  InitialOutput=0
  R_HC : Outport  Port=9  InitialOutput=0
  TR : Outport  Port=10  InitialOutput=0
  wires:
  [tr_mix] -> cal_torque/Trigger
  cal_torque/1(Torque) -> TR/1
  Energy_Int/1(E_mech) -> cal_torque/1(E_mech)
  crank/5(VT) -> [VT]
  [VT] -> frame/3(VT)
  frame/7(Qmax) -> knock_Integral/3(Qmax)
  ramining ratio of fuel/1(r_HC) -> R_HC/1
  [rad] -> ramining ratio of fuel/1(rad)
  knock_Integral/2(ki1) -> Knock/1
  [rps] -> knock_Integral/5(rps)
  frame/5(QA) -> knock_Integral/6(QA), ramining ratio of fuel/2(QA), QA/1
  [rad] -> knock_Integral/4(rad)
  EGR/1 -> frame/9(EGR)
  knock_Integral/1(ki) -> KI/1
  frame/4(QR) -> QR/1
  KL/1 -> frame/8(KL)
  [SA] -> frame/4(SA)
  crank/4(SA) -> [SA]
  Energy_Int/2(E) -> cal_cyl_state/1(E)
  cal_cyl_state/2(tc) -> heat_trans/3(tc), knock_Integral/2(Tc)
  cal_cyl_state/3(vol) -> heat_trans/4(vol)
  cal_cyl_state/4(cyl_st) -> cyl_state/1
  [rad] -> cal_cyl_state/4(rad)
  cal_cyl_state/1(pc) -> knock_Integral/1(pc), pc/1, Energy_Int/1(p), heat_trans/2(pc)
  crank/3(tr_inc) -> [tr_inc]
  cyl_conc/2(mix_mol) -> unburnt_gass/6(mix_mol)
  [tr_inc] -> frame/5(tr_inc)
  crank/6(Nfuel) -> unburnt_gass/1(Nfuel)
  frame/6(af) -> frame/7(AF), af/1
  crank/2(rad) -> [rad]
  [tr_mix] -> burnt_gass/2(tr_mix)
  [tr_mix] -> unburnt_gass/5(trig_mix)
  crank/1(trig_mix) -> [tr_mix]
  frame/1(burning gas) -> unburnt_gass/2(burning)
  ex_fml/1 -> unburnt_gass/4(gas_out)
  in_fen/1 -> Energy_Int/4(e_in)
  ex_fen/1 -> Energy_Int/3(e_out)
  [rad] -> frame/2(rad)
  [rad] -> Energy_Int/5(rad)
  ecu/1 -> crank/1(ecu)
  [rps] -> heat_trans/1(rps)
  cyl_conc/1(cyl_conc) -> cyl_c/1
  burnt_gass/1(mol_bs) -> cyl_conc/1(mol_bs), cal_cyl_state/3(mol_b)
  in_fml/1 -> unburnt_gass/3(gas_in)
  rps/1 -> Energy_Int/6(rps), frame/1(rps), [rps]
  unburnt_gass/1(mol_us) -> frame/6(mol_s), cal_cyl_state/2(mol_u), cyl_conc/2(mol_us)
  frame/3(burnt_gas) -> burnt_gass/1(gas_in)
  frame/2(q) -> Energy_Int/7(q)
  heat_trans/1(qw) -> Energy_Int/2(qw)

== system benchmark_model_2/ENGINE/engine_s/cylinders/cyl4/ex_valve ==
  d_st : Inport
  d_c : Inport  Port=2
  ecu : Inport  Port=3
  u_st : Inport  Port=4  PortDimensions=4
  u_c : Inport  Port=5
  Constant : Constant  Value=WOM
  Constant1 : Constant  Value=4*pi
  Gain : Gain  Gain=180/pi
  Lookup Table1 : Lookup  InputValues=THEX  Table=VAREX
  Math Function : Math  Operator=mod  SignedPower=on  SaturateOnIntegerOverflow=on
  Selector : Selector  InputPortWidth=6  IndexOptions=Index vector (dialog)  Indices=1  OutputSizes=[(-2)]
  cal_flow : MATLAB Function  TreatAsAtomicUnit=on
  fen : Outport  PortDimensions=1
  fml : Outport  Port=2  PortDimensions=7
  wires:
  Constant1/1 -> Math Function/2
  Selector/1 -> Math Function/1
  Math Function/1 -> Gain/1
  Gain/1 -> Lookup Table1/1
  Constant/1 -> cal_flow/6(WOM)
  cal_flow/2(fml) -> fml/1
  d_c/1 -> cal_flow/5(c_out)
  d_st/1 -> cal_flow/4(outlet)
  u_c/1 -> cal_flow/3(c_in)
  u_st/1 -> cal_flow/2(inlet)
  Lookup Table1/1 -> cal_flow/1(area)
  cal_flow/1(fen) -> fen/1
  ecu/1 -> Selector/1

== system benchmark_model_2/ENGINE/engine_s/cylinders/cyl4/in_valve ==
  d_c : Inport
  d_st : Inport  Port=2
  ecu : Inport  Port=3
  in_vt : Inport  Port=4
  u_st : Inport  Port=5
  u_c : Inport  Port=6
  Add : Sum  Inputs=-+
  Constant : Constant  Value=WOM
  Gain : Gain  Gain=180/pi
  Lookup Table : Lookup  InputValues=THIN  Table=VARIN
  Selector1 : Selector  InputPortWidth=6  IndexOptions=Index vector (dialog)  Indices=1  OutputSizes=[(-2)]
  cal_flow : MATLAB Function  TreatAsAtomicUnit=on
  fen : Outport  PortDimensions=1
  fml : Outport  Port=2  PortDimensions=7
  fms : Outport  Port=3  PortDimensions=1
  wires:
  Add/1 -> Gain/1
  Selector1/1 -> Add/2
  in_vt/1 -> Add/1
  Constant/1 -> cal_flow/6(WOM)
  cal_flow/3(fms) -> fms/1
  cal_flow/2(fml) -> fml/1
  d_c/1 -> cal_flow/5(c_out)
  u_c/1 -> cal_flow/3(c_in)
  cal_flow/1(fen) -> fen/1
  d_st/1 -> cal_flow/4(outlet)
  Lookup Table/1 -> cal_flow/1(area)
  u_st/1 -> cal_flow/2(inlet)
  ecu/1 -> Selector1/1
  Gain/1 -> Lookup Table/1

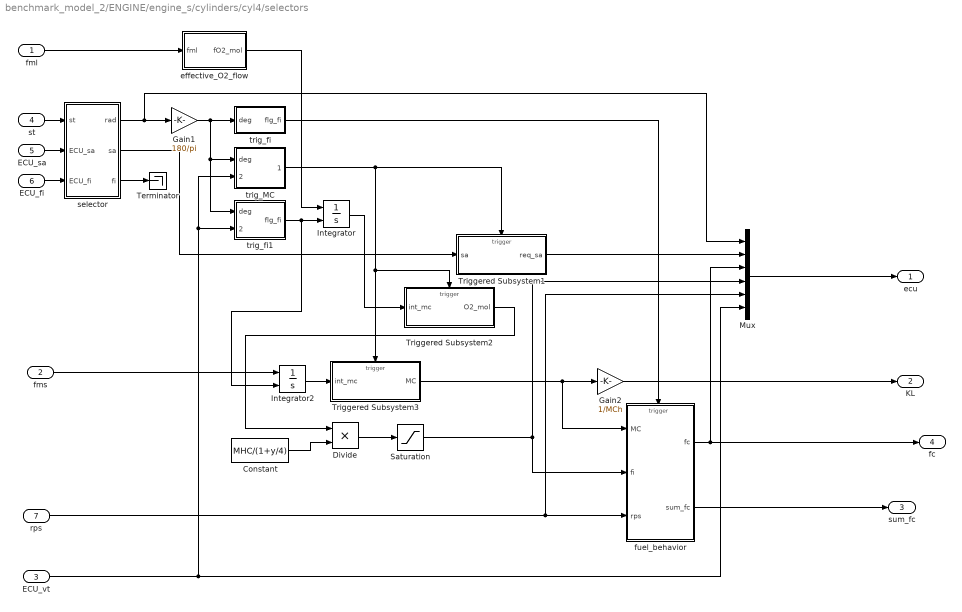
== system benchmark_model_2/ENGINE/engine_s/cylinders/cyl4/selectors ==
  fml : Inport
  fms : Inport  Port=2
  ECU_vt : Inport  Port=3
  st : Inport  Port=4
  ECU_sa : Inport  Port=5
  ECU_fi : Inport  Port=6
  rps : Inport  Port=7
  Constant : Constant  Value=MHC/(1+y/4)
  Divide : Product
  Gain1 : Gain  Gain=180/pi
  Gain2 : Gain  Gain=1/MCh
  Integrator : Integrator  ExternalReset=rising
  Integrator2 : Integrator  ExternalReset=rising
  Mux : Mux  Inputs=6
  Saturation : Saturate  UpperLimit=inf  LowerLimit=0
  Terminator : Terminator
  Triggered Subsystem1 : Subsystem  TreatAsAtomicUnit=on
  Triggered Subsystem2 : Subsystem  TreatAsAtomicUnit=on
  Triggered Subsystem3 : Subsystem  TreatAsAtomicUnit=on
  effective_O2_flow : Subsystem
  fuel_behavior : Subsystem  TreatAsAtomicUnit=on
  selector : Subsystem
  trig_MC : Subsystem
  trig_fi : Subsystem
  trig_fi1 : Subsystem
  ecu : Outport
  KL : Outport  Port=2
  sum_fc : Outport  Port=3
  fc : Outport  Port=4
  wires:
  fuel_behavior/2(sum_fc) -> sum_fc/1
  ECU_vt/1 -> Mux/6, trig_fi1/2(ECU_vvt), trig_MC/2(ECU_vvt)
  fms/1 -> Integrator2/1
  Triggered Subsystem3/1(MC) -> fuel_behavior/1(MC), Gain2/1
  Integrator2/1 -> Triggered Subsystem3/1(int_mc)
  Saturation/1 -> Mux/4, fuel_behavior/2(fi)
  Constant/1 -> Divide/2
  effective_O2_flow/1(fO2_mol) -> Integrator/1
  fml/1 -> effective_O2_flow/1(fml)
  Divide/1 -> Saturation/1
  Gain2/1 -> KL/1
  selector/3(fi) -> Terminator/1
  Integrator/1 -> Triggered Subsystem2/1(int_mc)
  trig_fi1/1(flg_fi) -> Integrator2/2, Integrator/2
  Triggered Subsystem1/1(req_sa) -> Mux/2
  selector/2(sa) -> Triggered Subsystem1/1(sa)
  trig_fi/1(flg_fi) -> fuel_behavior/Trigger
  Mux/1 -> ecu/1
  selector/1(rad) -> Mux/1, Gain1/1
  rps/1 -> fuel_behavior/3(rps), Mux/5
  trig_MC/1(flg_inc) -> Triggered Subsystem1/Trigger, Triggered Subsystem2/Trigger, Triggered Subsystem3/Trigger
  st/1 -> selector/1(st)
  ECU_sa/1 -> selector/2(ECU_sa)
  ECU_fi/1 -> selector/3(ECU_fi)
  Gain1/1 -> trig_MC/1(deg), trig_fi1/1(deg), trig_fi/1(deg)
  Triggered Subsystem2/1(O2_mol) -> Divide/1
  fuel_behavior/1(fc) -> fc/1, Mux/3

== system benchmark_model_2/ENGINE/engine_s/ex_chamber/In_vol/Enrgy_Int ==
  temp : Inport
  Enrgy_In : Inport  Port=2
  Enrgy_out : Inport  Port=3
  Enrgy_EGR : Inport  Port=4
  Constant1 : Constant  Value=TM0
  Gain : Gain  Gain=EX_M_AR*KET
  Sum : Sum  Inputs=-+--  InputSameDT=on  SaturateOnIntegerOverflow=on  OutDataTypeStr=Inherit: Same as first input
  Sum1 : Sum  Inputs=+-  InputSameDT=on  SaturateOnIntegerOverflow=on  OutDataTypeStr=Inherit: Same as first input
  energy_int : Integrator  InitialCondition=Einit
  E : Outport  InitialOutput=0
  wires:
  Gain/1 -> Sum/1
  Sum1/1 -> Gain/1
  Constant1/1 -> Sum1/2
  temp/1 -> Sum1/1
  Enrgy_In/1 -> Sum/2
  Enrgy_out/1 -> Sum/3
  Sum/1 -> energy_int/1
  energy_int/1 -> E/1
  Enrgy_EGR/1 -> Sum/4

== system benchmark_model_2/ENGINE/engine_s/ex_chamber/In_vol/Mol_Int ==
  nml_In : Inport
  nml_out : Inport  Port=2
  nml_EGR : Inport  Port=3
  Mol_Int : Integrator  InitialCondition=Ninit
  Sum : Sum  Inputs=+--  InputSameDT=on  SaturateOnIntegerOverflow=on  OutDataTypeStr=Inherit: Same as first input
  Nmol : Outport  InitialOutput=0
  wires:
  nml_In/1 -> Sum/1
  nml_out/1 -> Sum/2
  Sum/1 -> Mol_Int/1
  Mol_Int/1 -> Nmol/1
  nml_EGR/1 -> Sum/3

== system benchmark_model_2/ENGINE/engine_s/ex_chamber/In_vol/cal_cyl_state ==
  E : Inport
  Nml : Inport  Port=2
  Constant : Constant  Value=VL
  Divide : Product  Inputs=*/
  Dot Product : DotProduct  InputSameDT=on  OutDataTypeStr=Inherit: Inherit via internal rule
  Dot Product1 : DotProduct  InputSameDT=on  OutDataTypeStr=Inherit: Inherit via internal rule
  Sum of Elements : Sum  Inputs=+
  cal_state : Subsystem
  freedom : Constant  Value=FOM
  weight_mol : Constant  Value=WOM
  V_temp : Outport  InitialOutput=0
  V_st : Outport  Port=2  InitialOutput=0
  V_c : Outport  Port=3  InitialOutput=0
  wires:
  cal_state/2(ex_temp) -> V_temp/1
  Sum of Elements/1 -> cal_state/2(n), Divide/2
  freedom/1 -> Dot Product1/2
  Nml/1 -> Sum of Elements/1, Dot Product/2, Dot Product1/1, Divide/1
  weight_mol/1 -> Dot Product/1
  cal_state/1(ex_st) -> V_st/1
  Constant/1 -> cal_state/5(vol)
  E/1 -> cal_state/4(E)
  Divide/1 -> V_c/1
  Dot Product/1 -> cal_state/1(m)
  Dot Product1/1 -> cal_state/3(f)

== system benchmark_model_2/ENGINE/engine_s/in_chamber/In_vol/Enrgy_Int ==
  Enrgy_In : Inport
  Enrgy_out : Inport  Port=2
  Enrgy_EGR : Inport  Port=3
  Mass_Int : Integrator  InitialCondition=Einit
  Sum : Sum  Inputs=++-  InputSameDT=on  SaturateOnIntegerOverflow=on  OutDataTypeStr=Inherit: Same as first input
  X_dens : Outport  InitialOutput=0
  wires:
  Mass_Int/1 -> X_dens/1
  Sum/1 -> Mass_Int/1
  Enrgy_In/1 -> Sum/2
  Enrgy_out/1 -> Sum/3
  Enrgy_EGR/1 -> Sum/1

== system benchmark_model_2/ENGINE/engine_s/in_chamber/In_vol/Mol_Int ==
  nml_In : Inport
  nml_out : Inport  Port=2
  nml_EGR : Inport  Port=3
  Divide : Product  Inputs=/*
  Divide1 : Product  Inputs=*/
  Mol_Int : Integrator  InitialCondition=Ninit
  Sum : Sum  Inputs=++-  InputSameDT=on  SaturateOnIntegerOverflow=on  OutDataTypeStr=Inherit: Same as first input
  Sum of Elements : Sum  Inputs=+
  signiture_EGR : Subsystem
  signiture_EGR1 : Subsystem
  signiture_EGR2 : Subsystem
  signiture_EGR3 : Subsystem
  signiture_EGR4 : Subsystem
  Nmol : Outport  InitialOutput=0
  C_signed_C : Outport  Port=2  InitialOutput=0
  C_C : Outport  Port=3  InitialOutput=0
  wires:
  Sum/1 -> Mol_Int/1
  nml_In/1 -> signiture_EGR1/1(In)
  nml_out/1 -> signiture_EGR2/1(In)
  nml_EGR/1 -> signiture_EGR/1(In)
  signiture_EGR/1(Out) -> Sum/1
  signiture_EGR1/1(Out) -> Sum/2
  signiture_EGR2/1(Out) -> Sum/3
  Mol_Int/1 -> signiture_EGR3/1(In)
  signiture_EGR3/1(Out) -> Nmol/1, Sum of Elements/1, signiture_EGR4/1(In)
  Sum of Elements/1 -> Divide/1, Divide1/2
  signiture_EGR3/2(signed_C) -> Divide/2
  Divide/1 -> C_signed_C/1, signiture_EGR2/2(C_signed_C)
  Divide1/1 -> C_C/1
  signiture_EGR4/1(Out) -> Divide1/1

== system benchmark_model_2/ENGINE/engine_s/in_chamber/In_vol/cal_cyl_state ==
  E : Inport
  Nml : Inport  Port=2
  Constant : Constant  Value=VL
  Divide : Product  Inputs=*/
  Dot Product1 : DotProduct  InputSameDT=on  OutDataTypeStr=Inherit: Inherit via internal rule
  Dot Product2 : DotProduct  InputSameDT=on  OutDataTypeStr=Inherit: Inherit via internal rule
  Sum of Elements : Sum  Inputs=+
  cal_state : Subsystem
  freedom : Constant  Value=FOM
  weight_mol : Constant  Value=WOM
  V_st : Outport  InitialOutput=0
  V_c : Outport  Port=2  InitialOutput=0
  wires:
  Divide/1 -> V_c/1
  E/1 -> cal_state/4(E)
  Constant/1 -> cal_state/5(vol)
  cal_state/1(cyl_st) -> V_st/1
  Nml/1 -> Divide/1, Sum of Elements/1, Dot Product1/2, Dot Product2/1
  Sum of Elements/1 -> Divide/2, cal_state/2(n)
  Dot Product1/1 -> cal_state/1(m)
  weight_mol/1 -> Dot Product1/1
  Dot Product2/1 -> cal_state/3(f)
  freedom/1 -> Dot Product2/2

== system benchmark_model_2/ENGINE/engine_s/rpm_dynamics1/stroke/mod720(u,4*pi) ==
  u : Inport
  Constant7 : Constant  Value=4*pi
  Math Function : Math  Operator=mod  SignedPower=on  SaturateOnIntegerOverflow=on
  y : Outport
  wires:
  Constant7/1 -> Math Function/2
  u/1 -> Math Function/1
  Math Function/1 -> y/1

== system benchmark_model_2/ENGINE/engine_s/rpm_dynamics1/stroke/mod720(u,4*pi)1 ==
  u : Inport
  Constant7 : Constant  Value=4*pi
  Math Function : Math  Operator=mod  SignedPower=on  SaturateOnIntegerOverflow=on
  y : Outport
  wires:
  Math Function/1 -> y/1
  u/1 -> Math Function/1
  Constant7/1 -> Math Function/2

== system benchmark_model_2/ENGINE/engine_s/rpm_dynamics1/stroke/mod720(u,4*pi)2 ==
  u : Inport
  Constant7 : Constant  Value=4*pi
  Math Function : Math  Operator=mod  SignedPower=on  SaturateOnIntegerOverflow=on
  y : Outport
  wires:
  Constant7/1 -> Math Function/2
  u/1 -> Math Function/1
  Math Function/1 -> y/1

== system benchmark_model_2/ENGINE/engine_s/rpm_dynamics1/stroke/mod720(u,4*pi)3 ==
  u : Inport
  Constant7 : Constant  Value=4*pi
  Math Function : Math  Operator=mod  SignedPower=on  SaturateOnIntegerOverflow=on
  y : Outport
  wires:
  Math Function/1 -> y/1
  u/1 -> Math Function/1
  Constant7/1 -> Math Function/2

== system benchmark_model_2/ENGINE/engine_s/cylinders/cyl1/cyl/Energy_Int ==
  p : Inport
  qw : Inport  Port=2
  e_out : Inport  Port=3
  e_in : Inport  Port=4
  rad : Inport  Port=5
  rps : Inport  Port=6
  q : Inport  Port=7
  Constant : Constant  Value=PR0
  Product : Product  RndMeth=Zero
  Product1 : Product  RndMeth=Zero
  Subtract : Sum  Inputs=+-
  Sum2 : Sum  Inputs=+--+-  InputSameDT=on  SaturateOnIntegerOverflow=on  OutDataTypeStr=Inherit: Same as first input
  dvol : Subsystem
  int_e : Integrator  InitialCondition=(FD0/2.0)*PR0*VT
  int_pdv : Integrator
  E_mech : Outport  InitialOutput=0
  E : Outport  Port=2  InitialOutput=0
  wires:
  qw/1 -> Sum2/2
  e_out/1 -> Sum2/3
  Product/1 -> Sum2/5
  e_in/1 -> Sum2/4
  q/1 -> Sum2/1
  int_e/1 -> E/1
  Sum2/1 -> int_e/1
  rad/1 -> dvol/1(rad)
  dvol/1(dvol) -> Product1/1, Product/2
  rps/1 -> dvol/2(rps)
  int_pdv/1 -> E_mech/1
  p/1 -> Subtract/1, Product/1
  Constant/1 -> Subtract/2
  Subtract/1 -> Product1/2
  Product1/1 -> int_pdv/1

== system benchmark_model_2/ENGINE/engine_s/cylinders/cyl1/cyl/burnt_gass ==
  gas_in : Inport
  tr_mix : Inport  Port=2
  Mass_Int : Integrator  ExternalReset=rising  InitialCondition=[0;0;0;0;0;0;0]
  Memory2 : Memory
  mol_bs : Outport  PortDimensions=7  InitialOutput=0
  wires:
  Mass_Int/1 -> mol_bs/1
  gas_in/1 -> Mass_Int/1
  tr_mix/1 -> Memory2/1
  Memory2/1 -> Mass_Int/2

== system benchmark_model_2/ENGINE/engine_s/cylinders/cyl1/cyl/cal_cyl_state ==
  E : Inport
  mol_u : Inport  Port=2
  mol_b : Inport  Port=3
  rad : Inport  Port=4
  Add2 : Sum
  Constant : Constant  Value=SPEC
  Dot Product2 : DotProduct  InputSameDT=on  OutDataTypeStr=Inherit: Inherit via internal rule
  Dot Product3 : DotProduct  InputSameDT=on  OutDataTypeStr=Inherit: Inherit via internal rule
  Sum of Elements : Sum  Inputs=+
  cal_state : Subsystem
  cyl_vol : MATLAB Function  TreatAsAtomicUnit=on
  freedom : Constant  Value=FOM
  weight_mol : Constant  Value=WOM
  pc : Outport  InitialOutput=0
  tc : Outport  Port=2  InitialOutput=0
  vol : Outport  Port=3  InitialOutput=0
  cyl_st : Outport  Port=4  InitialOutput=0
  wires:
  E/1 -> cal_state/4(E)
  rad/1 -> cyl_vol/1(u)
  Constant/1 -> cyl_vol/2(SPEC)
  cal_state/1(pc) -> pc/1
  cal_state/2(tc) -> tc/1
  cal_state/3(cyl_st) -> cyl_st/1
  cyl_vol/1(vol) -> vol/1, cal_state/5(vol)
  weight_mol/1 -> Dot Product2/1
  mol_b/1 -> Add2/1
  mol_u/1 -> Add2/2
  Add2/1 -> Sum of Elements/1, Dot Product2/2, Dot Product3/1
  freedom/1 -> Dot Product3/2
  Sum of Elements/1 -> cal_state/2(n)
  Dot Product2/1 -> cal_state/1(m)
  Dot Product3/1 -> cal_state/3(f)

== system benchmark_model_2/ENGINE/engine_s/cylinders/cyl1/cyl/cal_torque ==
  E_mech : Inport
  Trigger : TriggerPort  VariantControl=(inherit)  PortDimensions=1
  Constant : Constant  Value=4*pi
  Divide : Product  Inputs=*/
  Subtract : Sum  Inputs=+-
  Unit Delay : UnitDelay  SampleTime=-1  HasFrameUpgradeWarning=on
  Torque : Outport
  wires:
  Unit Delay/1 -> Subtract/2
  E_mech/1 -> Subtract/1, Unit Delay/1
  Subtract/1 -> Divide/1
  Divide/1 -> Torque/1
  Constant/1 -> Divide/2
